simulink model "TP2"  (Simulink 9.0)
settings: Solver=ode23t  StartTime=0.0  StopTime=2  RelTol=1e-3
InitFcn:
  | TD2_config
values from neighbouring files (symbols this model uses):
  b = 8.5E-3    (= 0.0085)    [TD2_config.m]    (also in TP2_config.m)
  J = 0.28    [TD2_config.m]    (also in TP2_config.m)
  K = 0.5093    [TD2_config.m]    (also in TP2_config.m)
  L = 1.6E-3    (= 0.0016)    [TD2_config.m]    (also in TP2_config.m)
  R = 0.13    [TD2_config.m]    (also in TP2_config.m)
libraries: simulink x2
settings Model: Creator=GEII Robot  LastModifiedBy=GEII Robot
settings DataIOCC: SaveFormat=Dataset
settings OptimizationCC: LifeSpan=auto
settings DebuggingCC: UnderspecifiedInitializationDetection=Simplified  MergeDetectMultiDrivingBlocksExec=error  SFUnexpectedBacktrackingDiag=error  SFNoUnconditionalDefaultTransitionDiag=error  SFExecutionAtInitializationDiag=warning
settings HardwareCC: ProdBitPerPointer=64  ProdBitPerSizeT=64  ProdBitPerPtrDiffT=64  ProdLargestAtomicFloat=Float  ProdIntDivRoundTo=Zero  ProdEndianess=LittleEndian  ProdWordSize=64  ProdHWDeviceType=Intel->x86-64 (Windows64)
settings ModelReferenceCC: PropagateSignalLabelsOutOfModel=on
settings CodeAppCC: StateflowObjectComments=off
settings GRTTargetCC: TargetLangStandard=C99 (ISO)
settings ConfigComp: CovMetricSettings=dwe  CovHtmlReporting=off  CovSaveCumulativeToWorkspaceVar=off  CovSaveSingleToWorkspaceVar=off  CovExternalEMLEnable=on

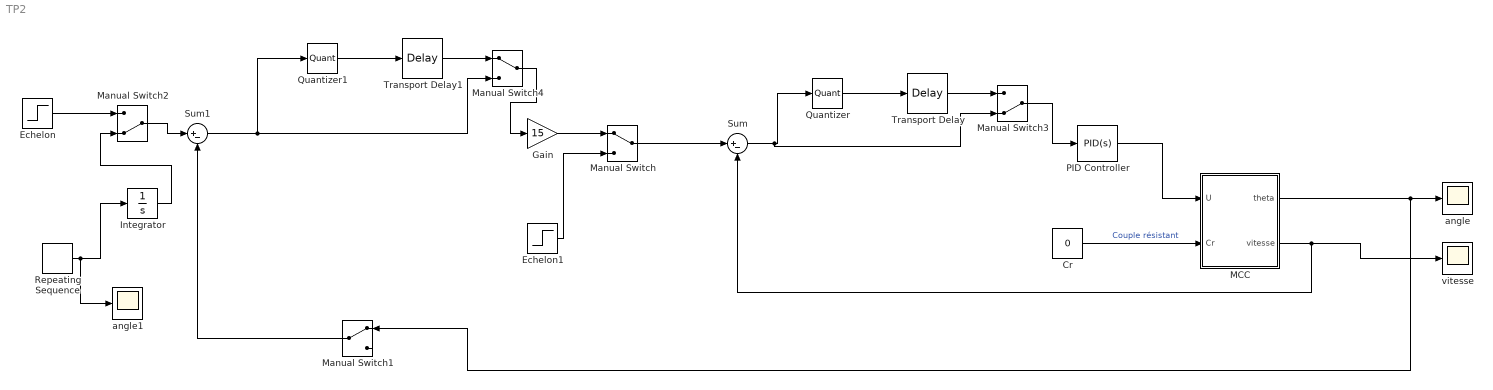
== system TP2 ==
  Cr : Constant  Value=0
  Echelon : Step  Time=0  SampleTime=0
  Echelon1 : Step  Time=0  SampleTime=0
  Gain : Gain  Gain=15
  Integrator : Integrator
  MCC : Subsystem
  Manual Switch : ManualSwitch
  Manual Switch1 : ManualSwitch
  Manual Switch2 : ManualSwitch  CurrentSetting=0
  Manual Switch3 : ManualSwitch  CurrentSetting=0
  Manual Switch4 : ManualSwitch
  PID Controller : simulink/Continuous/PID Controller  Controller=PID  TimeDomain=Continuous-time  SampleTime=-1  IntegratorMethod=Forward Euler  FilterMethod=Forward Euler  Form=Parallel  UseFilter=on  ControllerParametersSource=internal  P=3  I=25  D=0.02  N=100  InitialConditionSource=internal  InitialConditionForIntegrator=0  InitialConditionForFilter=0  ExternalReset=none  LimitOutput=off  UpperSaturationLimit=inf  LowerSaturationLimit=-inf  LinearizeAsGain=on  AntiWindupMode=none  Kb=1  TrackingMode=off  Kt=1  PParamMin=[]  PParamMax=[]  IParamMin=[]  IParamMax=[]  DParamMin=[]  DParamMax=[]  NParamMin=[]  NParamMax=[]  KbParamMin=[]  KbParamMax=[]  KtParamMin=[]  KtParamMax=[]  POutMin=[]  POutMax=[]  IOutMin=[]  IOutMax=[]  DOutMin=[]  DOutMax=[]  NOutMin=[]  NOutMax=[]  KbOutMin=[]  KbOutMax=[]  KtOutMin=[]  KtOutMax=[]  IntegratorOutMin=[]  IntegratorOutMax=[]  FilterOutMin=[]  FilterOutMax=[]  SumOutMin=[]  SumOutMax=[]  SumI1OutMin=[]  SumI1OutMax=[]  SumI2OutMin=[]  SumI2OutMax=[]  SumI3OutMin=[]  SumI3OutMax=[]  SumDOutMin=[]  SumDOutMax=[]  SaturationOutMin=[]  SaturationOutMax=[]  IntegratorContinuousStateAttributes=''  IntegratorStateMustResolveToSignalObject=off  IntegratorRTWStateStorageClass=Auto  FilterContinuousStateAttributes=''  FilterStateMustResolveToSignalObject=off  FilterRTWStateStorageClass=Auto  DifferentiatorICPrevScaledInput=0  DifferentiatorOutMin=[]  DifferentiatorOutMax=[]  InitialConditionSetting=State (most efficient)  FilterDiffOutCoefMin=[]  FilterDiffOutCoefMax=[]  SumDenOutMin=[]  SumDenOutMax=[]  SumNumOutMin=[]  SumNumOutMax=[]  ReciprocalOutMin=[]  ReciprocalOutMax=[]  DivideOutMin=[]  DivideOutMax=[]  TunerSelectOption=Transfer Function Based (PID Tuner App)
  Quantizer : Quantizer  QuantizationInterval=0.02
  Quantizer1 : Quantizer  QuantizationInterval=0.02
  Repeating Sequence : simulink/Sources/Repeating Sequence  rep_seq_t=[0 0.2 0.25 0.3 0.5]  rep_seq_y=[0 50 50 0 0]
  Sum : Sum  Inputs=|+-
  Sum1 : Sum  Inputs=|+-
  Transport Delay : TransportDelay  DelayTime=0.1
  Transport Delay1 : TransportDelay  DelayTime=0
  angle : Scope
  angle1 : Scope
  vitesse : Scope
  wires:
  Cr/1 -> MCC/2(Cr)  "Couple résistant"
  MCC/1(theta) -> Manual Switch1/1, angle/1
  MCC/2(vitesse) -> Sum/2, vitesse/1
  PID Controller/1 -> MCC/1(U)
  Gain/1 -> Manual Switch/1
  Manual Switch/1 -> Sum/1
  Echelon1/1 -> Manual Switch/2
  Manual Switch1/1 -> Sum1/2
  Repeating Sequence/1 -> angle1/1, Integrator/1
  Integrator/1 -> Manual Switch2/2
  Manual Switch2/1 -> Sum1/1
  Echelon/1 -> Manual Switch2/1
  Quantizer/1 -> Transport Delay/1
  Sum/1 -> Manual Switch3/2, Quantizer/1
  Transport Delay/1 -> Manual Switch3/1
  Manual Switch3/1 -> PID Controller/1
  Transport Delay1/1 -> Manual Switch4/1
  Quantizer1/1 -> Transport Delay1/1
  Sum1/1 -> Manual Switch4/2, Quantizer1/1
  Manual Switch4/1 -> Gain/1

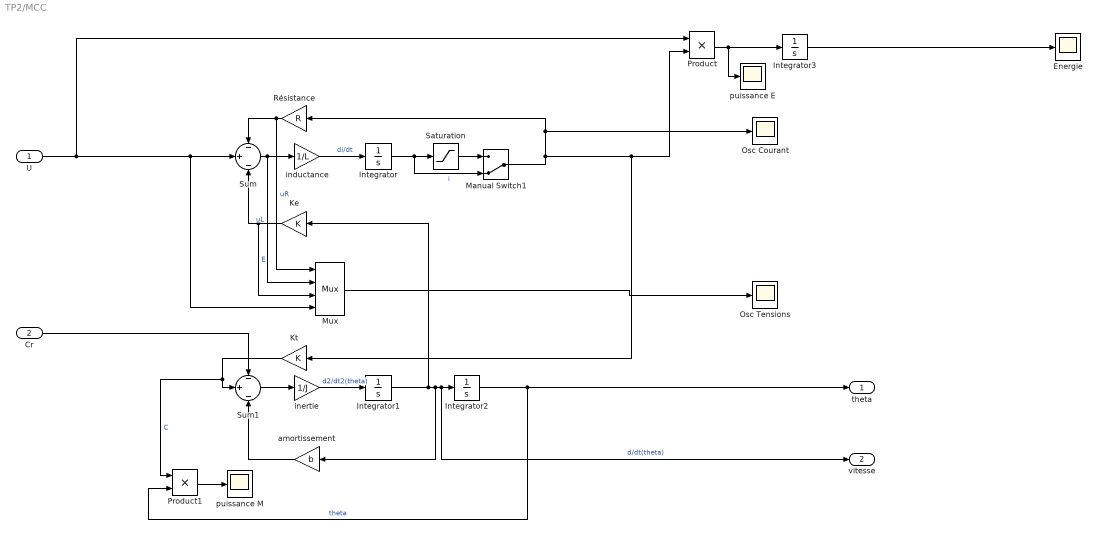
== system TP2/MCC ==
  U : Inport
  Cr : Inport  Port=2
  Energie : Scope
  Integrator{,1..3} (4 alike) : Integrator
  Ke : Gain  Gain=K
  Kt : Gain  Gain=K
  Manual Switch1 : ManualSwitch  CurrentSetting=0
  Mux : Mux
      settings: DisplayOption=signals
  "Osc Courant " : Scope
  Osc Tensions : Scope
  Product : Product
  Product1 : Product
  Résistance : Gain  Gain=R
  Saturation : Saturate  UpperLimit=20  LowerLimit=-20
  Sum : Sum  Inputs=-|+|-
  Sum1 : Sum  Inputs=-|+|-
  amortissement : Gain  Gain=b
  inductance : Gain  Gain=1/L
  inertie : Gain  Gain=1/J
  puissance E : Scope
  puissance M : Scope
  theta : Outport
  vitesse : Outport  Port=2
  wires:
  Cr/1 -> Sum1/1
  amortissement/1 -> Sum1/3
  Résistance/1 -> Mux/1, Sum/1  "uR"
  Integrator2/1 -> Product1/2, theta/1  "theta"
  Ke/1 -> Mux/3, Sum/3  "E"
  U/1 -> Product/1, Mux/4, Sum/2
  Integrator1/1 -> Ke/1, amortissement/1, vitesse/1, Integrator2/1  "d/dt(theta)"
  Kt/1 -> Product1/1, Sum1/2  "C"
  Sum/1 -> Mux/2, inductance/1  "uL"
  inductance/1 -> Integrator/1  "di/dt"
  Mux/1 -> Osc Tensions/1
  inertie/1 -> Integrator1/1  "d2/dt2(theta)"
  Sum1/1 -> inertie/1
  Product/1 -> puissance E/1, Integrator3/1
  Integrator3/1 -> Energie/1
  Product1/1 -> puissance M/1
  Manual Switch1/1 -> Résistance/1, "Osc Courant "/1, Product/2, Kt/1
  Integrator/1 -> Manual Switch1/2, Saturation/1  "i"
  Saturation/1 -> Manual Switch1/1
